simulink model "GridFormingConverter"  (R2023a)
settings: Solver=ode1be  StartTime=0.0  StopTime=simulationTime  FixedStep=gridInverter.vsm.samplingTime  MaxStep=gridInverter.vsm.samplingTime  RelTol=1e-3  AbsTol=1e-3
PreLoadFcn:
  | % Parameterize the model
  | GridFormingConverterInputParameters;
PostLoadFcn:
  | GridFormingConverterTestCondition;
undefined symbols (not defined in the file): base, DiscIntNeverNeededParam, grid, gridInverter, localSolverSampleTime, scrFactorRg, scrFactorXg, transformer, TransmissionLine
libraries: ee_lib x15, eeGeneralControl x15, nesl_utility x11, simulink x5, fl_lib x4, eeTransforms x4, eeSinGeneratorThreePhase x1, simulink_extras x1, eePowerMeasurement x1
(part 2 of 3)

== system GridFormingConverter/Grid-Forming Converter/Grid-Forming Converter Control/Current Limiting ==
  In Bus Element : Inport  PortName=measure  Element=Igd
  In Bus Element1 : Inport  PortName=measure  Element=Igq
  In Bus Element2 : Inport  Port=2  PortName=reactiveControl  Element=Vmd
  In Bus Element4 : Inport  Port=2  PortName=reactiveControl  Element=Vmq
  CurrentLimitingMethod : Subsystem  Variant=on  VariantControlMode=label  VariantControl=Choice  LabelModeActiveChoice=virimp
  Subtract : Sum  Inputs=+-
  Subtract1 : Sum  Inputs=-+
  Out Bus Element : Outport  PortName=currentLimiting  Element=Vmd
  Out Bus Element1 : Outport  PortName=currentLimiting  Element=Vmq
  Out Bus Element2 : Outport  PortName=currentLimiting  Element=Idmax
  Out Bus Element3 : Outport  PortName=currentLimiting  Element=Iqmax
  wires:
  In Bus Element2/1 -> Subtract/1
  In Bus Element1/1 -> CurrentLimitingMethod/2(Igq)
  In Bus Element4/1 -> Subtract1/2
  Subtract/1 -> Out Bus Element/1
  Subtract1/1 -> Out Bus Element1/1
  In Bus Element/1 -> CurrentLimitingMethod/1(Igd)  "Q"
  CurrentLimitingMethod/1(delVd) -> Subtract/2
  CurrentLimitingMethod/2(delVq) -> Subtract1/1
  CurrentLimitingMethod/3(Idmax) -> Out Bus Element2/1
  CurrentLimitingMethod/4(Iqmax) -> Out Bus Element3/1

== system GridFormingConverter/Grid-Forming Converter/Grid-Forming Converter Control/Grid Voltage Reactive Power Support ==
  In Bus Element1 : Inport  PortName=measure  Element=Vgd
  In Bus Element3 : Inport  PortName=measure  Element=Vgq
  In Bus Element2 : Inport  PortName=measure  Element=Igd
  In Bus Element4 : Inport  PortName=measure  Element=Igq
  PrefInput : Inport  Port=2
  QrefInput : Inport  Port=3
  Modifying Active Power Reference : Subsystem
  Modifying Reactive Power Reference : Subsystem
  Rate Transition{,1..5} (6 alike) : RateTransition
  Pref : Outport
  Qref : Outport  Port=2
  wires:
  PrefInput/1 -> Modifying Active Power Reference/1(PrefInput)
  In Bus Element2/1 -> Modifying Active Power Reference/3(Igd)
  In Bus Element4/1 -> Modifying Active Power Reference/4(Igq)
  In Bus Element3/1 -> Rate Transition2/1
  QrefInput/1 -> Rate Transition3/1
  Modifying Reactive Power Reference/1(PrefNew) -> Rate Transition4/1
  Modifying Reactive Power Reference/2(QrefNew) -> Rate Transition5/1
  In Bus Element1/1 -> Rate Transition/1
  Modifying Active Power Reference/1(Pref) -> Rate Transition1/1
  Rate Transition2/1 -> Modifying Reactive Power Reference/2(Vgq)
  Rate Transition3/1 -> Modifying Reactive Power Reference/3(Qref)
  Rate Transition1/1 -> Modifying Reactive Power Reference/4(Pref)
  Rate Transition4/1 -> Pref/1
  Rate Transition5/1 -> Qref/1
  Rate Transition/1 -> Modifying Reactive Power Reference/1(Vgd), Modifying Active Power Reference/2(Vd)

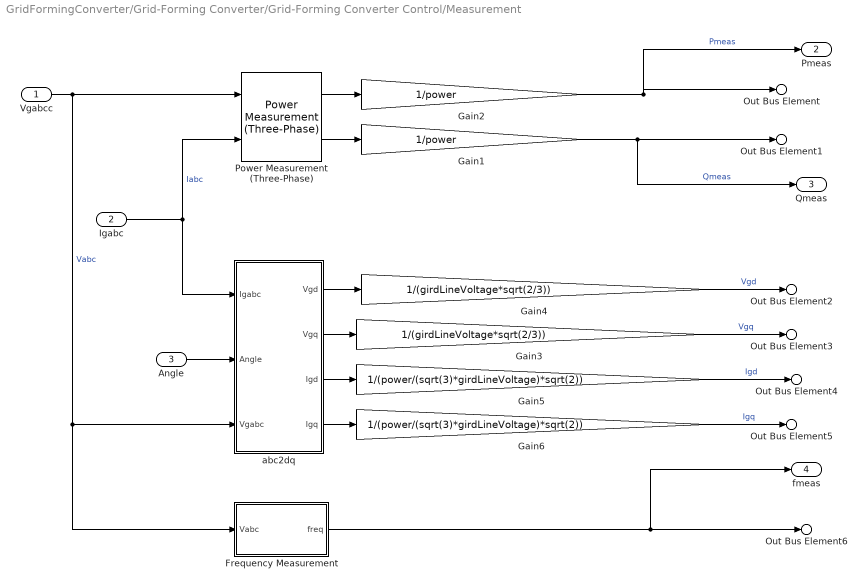
== system GridFormingConverter/Grid-Forming Converter/Grid-Forming Converter Control/Measurement ==
  Vgabcc : Inport
  Igabc : Inport  Port=2
  Angle : Inport  Port=3
  Frequency Measurement : Subsystem
  Gain1 : Gain  Gain=1/power
  Gain2 : Gain  Gain=1/power
  Gain3 : Gain  Gain=1/(girdLineVoltage*sqrt(2/3))
  Gain4 : Gain  Gain=1/(girdLineVoltage*sqrt(2/3))
  Gain5 : Gain  Gain=1/(power/(sqrt(3)*girdLineVoltage)*sqrt(2))
  Gain6 : Gain  Gain=1/(power/(sqrt(3)*girdLineVoltage)*sqrt(2))
  Power Measurement (Three-Phase) : eePowerMeasurement/Power Measurement (Three-Phase)  LabelModeActiveChoice=Continuous  F=powerFreq  K=[1]  Seq=Positive  Ts=measSampleTime
  abc2dq : Subsystem
  Out Bus Element : Outport  PortName=measure  Element=P
  Out Bus Element1 : Outport  PortName=measure  Element=Q
  Out Bus Element2 : Outport  PortName=measure  Element=Vgd
  Out Bus Element3 : Outport  PortName=measure  Element=Vgq
  Out Bus Element4 : Outport  PortName=measure  Element=Igd
  Out Bus Element5 : Outport  PortName=measure  Element=Igq
  Out Bus Element6 : Outport  PortName=measure  Element=fgrid
  Pmeas : Outport  Port=2
  Qmeas : Outport  Port=3
  fmeas : Outport  Port=4
  wires:
  Vgabcc/1 -> abc2dq/3(Vgabc), Frequency Measurement/1(Vabc), Power Measurement (Three-Phase)/1  "Vabc"
  Angle/1 -> abc2dq/2(Angle)
  Power Measurement (Three-Phase)/1 -> Gain2/1
  Igabc/1 -> abc2dq/1(Igabc), Power Measurement (Three-Phase)/2  "Iabc"
  Power Measurement (Three-Phase)/2 -> Gain1/1
  Gain2/1 -> Pmeas/1, Out Bus Element/1  "Pmeas"
  Gain1/1 -> Qmeas/1, Out Bus Element1/1  "Qmeas"
  abc2dq/1(Vgd) -> Gain4/1
  abc2dq/2(Vgq) -> Gain3/1
  abc2dq/3(Igd) -> Gain5/1
  abc2dq/4(Igq) -> Gain6/1
  Gain3/1 -> Out Bus Element3/1  "Vgq"
  Gain4/1 -> Out Bus Element2/1  "Vgd"
  Gain5/1 -> Out Bus Element4/1  "Igd"
  Gain6/1 -> Out Bus Element5/1  "Igq"
  Frequency Measurement/1(freq) -> Out Bus Element6/1, fmeas/1

== system GridFormingConverter/Grid-Forming Converter/Grid-Forming Converter Control/Power Control ==
  note: Reactive Power Control
  note: Active Power Control
  In Bus Element2 : Inport  PortName=measure  Element=P
  In Bus Element3 : Inport  PortName=measure  Element=Q
  In Bus Element1 : Inport  PortName=measure  Element=fgrid
  Pref : Inport  Port=2
  Qref : Inport  Port=3
  ActivePowerControl : Subsystem  Variant=on  VariantControlMode=label  VariantControl=Choice  LabelModeActiveChoice=vsm
  ReactiveControl : Subsystem
  Out Bus Element : Outport  PortName=reactiveControl  Element=Vmd
  Out Bus Element1 : Outport  PortName=reactiveControl  Element=Vmq
  Out Bus Element6 : Outport  Port=2  PortName=activeControl  Element=angle
  Out Bus Element4 : Outport  Port=2  PortName=activeControl  Element=w
  angle : Outport  Port=3
  wires:
  ActivePowerControl/2(w) -> Out Bus Element4/1
  In Bus Element3/1 -> ReactiveControl/2(Qmeas)
  ActivePowerControl/1(Theta) -> angle/1, Out Bus Element6/1
  ReactiveControl/1(Vmd) -> Out Bus Element/1
  ReactiveControl/2(Vmq) -> Out Bus Element1/1
  Pref/1 -> ActivePowerControl/1(Pref)  "Q"
  Qref/1 -> ReactiveControl/1(Qref)  "Q"
  In Bus Element2/1 -> ActivePowerControl/2(Pmeas)
  In Bus Element1/1 -> ActivePowerControl/3(fgrid)

== system GridFormingConverter/Grid-Forming Converter/Grid-Forming Converter Control/VoltageCurrentControl ==
  In Bus Element : Inport  PortName=currentLimiting  Element=Vmd
  In Bus Element1 : Inport  PortName=currentLimiting  Element=Vmq
  In Bus Element6 : Inport  PortName=currentLimiting  Element=Idmax
  In Bus Element7 : Inport  PortName=currentLimiting  Element=Iqmax
  Bus Element In6 : Inport  Port=2  PortName=activeControl  Element=w
  Bus Element In1 : Inport  Port=2  PortName=activeControl  Element=angle
  In Bus Element2 : Inport  Port=3  PortName=measure  Element=Vgd
  In Bus Element3 : Inport  Port=3  PortName=measure  Element=Vgq
  In Bus Element4 : Inport  Port=3  PortName=measure  Element=Igd
  In Bus Element5 : Inport  Port=3  PortName=measure  Element=Igq
  Controller : Subsystem
  Modulation Signal : Subsystem
  mabc : Outport
  wires:
  Controller/2(Vq) -> Modulation Signal/2(Vq)
  Modulation Signal/1(mabc) -> mabc/1
  Controller/1(Vd) -> Modulation Signal/1(Vd)
  In Bus Element4/1 -> Controller/6(Id)
  In Bus Element5/1 -> Controller/7(Iq)
  In Bus Element6/1 -> Controller/8(Idmax)
  In Bus Element7/1 -> Controller/9(Iqmax)
  In Bus Element2/1 -> Controller/4(Vsd)
  In Bus Element3/1 -> Controller/5(Vsq)
  Bus Element In6/1 -> Controller/1(Angfreq)
  In Bus Element/1 -> Controller/2(Vgdref)
  In Bus Element1/1 -> Controller/3(Vgqref)
  Bus Element In1/1 -> Modulation Signal/3(Angle)

== system GridFormingConverter/Grid-Forming Converter/Grid-Forming Converter Power Circuit/Filter & Sensor ==
  Current Sensor (Three-Phase) : ee_lib/Sensors & Transducers/Current Sensor (Three-Phase)
  Electrical Reference1 : fl_lib/Electrical/Electrical Elements/Electrical Reference
  Low-Pass Filter (Discrete or Continuous)1 : eeGeneralControl/Low-Pass Filter (Discrete or Continuous)  K=1  T=1/(200*gridInverter.frequency)  B=inf  A=-inf  init_option=Specify as parameter  x0=0  Ts=gridInverter.controller.VoltageControlSampleTime
  Low-Pass Filter (Discrete or Continuous)2 : eeGeneralControl/Low-Pass Filter (Discrete or Continuous)  K=1  T=1/(200*gridInverter.frequency)  B=inf  A=-inf  init_option=Specify as parameter  x0=0  Ts=gridInverter.controller.VoltageControlSampleTime
  Neutral Port (Three-Phase) : ee_lib/Connectors & References/Neutral Port (Three-Phase)  G_parasitic=1e-12 1/Ohm
      settings: InternalSimscapePortConfiguration="{\"Bottom\":[],\"Left\":[{\"id\":\"N\",\"label\":\"~\",\"type\":\"foundation.electrical.three_phase\"}],\"Right\":[{\"id\":\"n\",\"label\":\"n\",\"type\":\"foundation.electrical.electrical\"}],\"Top\":[]}"
  PS-Simulink Converter : nesl_utility/PS-Simulink Converter  PhysicalDomain=network_engine_domain  SubClassName=ps_output  LeftPortType=input  RightPortType=output  PseudoPeriodic=off  Frequencies=[]  VectorFormat=inherit  Unit=inherit  AffineConversion=off
  PS-Simulink Converter1 : nesl_utility/PS-Simulink Converter  PhysicalDomain=network_engine_domain  SubClassName=ps_output  LeftPortType=input  RightPortType=output  PseudoPeriodic=off  Frequencies=[]  VectorFormat=inherit  Unit=inherit  AffineConversion=off
  Phase Voltage Sensor (Three-Phase) : ee_lib/Sensors & Transducers/Phase Voltage Sensor (Three-Phase)
  RLC (Three-Phase) : ee_lib/Passive/RLC Assemblies/RLC (Three-Phase)  component_structure=ee.enum.rlc.structure.SeriesRL  R=gridInverter.lineResistance Ohm  L=gridInverter.L H  C=1e-6 F  R_parasitic=0 Ohm  G_parasitic=0 1/Ohm  IL_specify=off  IL_priority=High  IL=[0, 0, 0] A  IL_nominal_specify=off  IL_nominal_unit=A  IL_nominal_value=1  VC_specify=off  VC_priority=High  VC=[0, 0, 0] V  VC_nominal_specify=off  VC_nominal_unit=V  VC_nominal_value=1
      settings: InternalSimscapePortConfiguration="{\"Bottom\":[],\"Left\":[{\"id\":\"N1\",\"label\":\"~1\",\"type\":\"foundation.electrical.three_phase\"}],\"Right\":[{\"id\":\"N2\",\"label\":\"~2\",\"type\":\"foundation.electrical.three_phase\"}],\"Top\":[]}"
  Inabc : PMIOPort  Side=Left
  Opabc : PMIOPort  Port=2  Side=Right
  Iabc : Outport
  Vabc : Outport  Port=2
  wires:
  PS-Simulink Converter1/1 -> Low-Pass Filter (Discrete or Continuous)1/1
  Low-Pass Filter (Discrete or Continuous)2/1 -> Iabc/1
  PS-Simulink Converter/1 -> Low-Pass Filter (Discrete or Continuous)2/1
  Low-Pass Filter (Discrete or Continuous)1/1 -> Vabc/1
  connections:
  PS-Simulink Converter1/LConn1 -- Phase Voltage Sensor (Three-Phase)/RConn1
  Current Sensor (Three-Phase)/RConn2 -- RLC (Three-Phase)/LConn1
  Current Sensor (Three-Phase)/LConn1 -- Inabc/RConn1
  PS-Simulink Converter/LConn1 -- Current Sensor (Three-Phase)/RConn1
  Phase Voltage Sensor (Three-Phase)/LConn1 -- Opabc/RConn1 -- RLC (Three-Phase)/RConn1
  Phase Voltage Sensor (Three-Phase)/RConn2 -- Neutral Port (Three-Phase)/LConn1
  Electrical Reference1/LConn1 -- Neutral Port (Three-Phase)/RConn1

== system GridFormingConverter/Grid-Forming Converter/Grid-Forming Converter Control/Current Limiting/CurrentLimitingMethod ==
  Igd : Inport
  Igq : Inport  Port=2
  currentLimitAndVirtual : Subsystem  VariantControl=both
  currentSaturation : Subsystem  VariantControl=ctSat
  virtualImpedance : Subsystem  VariantControl=virimp
  delVd : Outport
  delVq : Outport  Port=2
  Idmax : Outport  Port=3
  Iqmax : Outport  Port=4

== system GridFormingConverter/Grid-Forming Converter/Grid-Forming Converter Control/Grid Voltage Reactive Power Support/Modifying Active Power Reference ==
  PrefInput : Inport
  Vd : Inport  Port=2
  Igd : Inport  Port=3
  Igq : Inport  Port=4
  AND : Logic  IconShape=distinctive  AllPortsSameDT=off  OutDataTypeStr=boolean
  Abs : Abs  SaturateOnIntegerOverflow=off
  Compare To Constant : simulink/Logic and Bit Operations/Compare To Constant  relop=<=  const=0.90  OutDataTypeStr=boolean
  Computing New Active Power Ref : Subsystem
  Math Function1 : Math  Operator=hypot
  Power Sign : Signum
  Product : Product
  Rate Transition1 : RateTransition
  Relay : Relay  OnSwitchValue=maxVICurrentLimit*0.96  OffSwitchValue=1
  Switch : Switch  Criteria=u2 > Threshold  SaturateOnIntegerOverflow=off  InputSameDT=off
  Pref : Outport
  wires:
  Computing New Active Power Ref/1(Pref) -> Switch/1
  Math Function1/1 -> Rate Transition1/1  "Is"
  Vd/1 -> Computing New Active Power Ref/2(Vd), Compare To Constant/1
  PrefInput/1 -> Power Sign/1, Switch/3
  Igd/1 -> Math Function1/2
  Switch/1 -> Abs/1
  Abs/1 -> Product/1
  Power Sign/1 -> Product/2
  Product/1 -> Pref/1
  Relay/1 -> AND/2
  AND/1 -> Switch/2
  Compare To Constant/1 -> AND/1
  Igq/1 -> Computing New Active Power Ref/1(Iq), Math Function1/1
  Rate Transition1/1 -> Relay/1

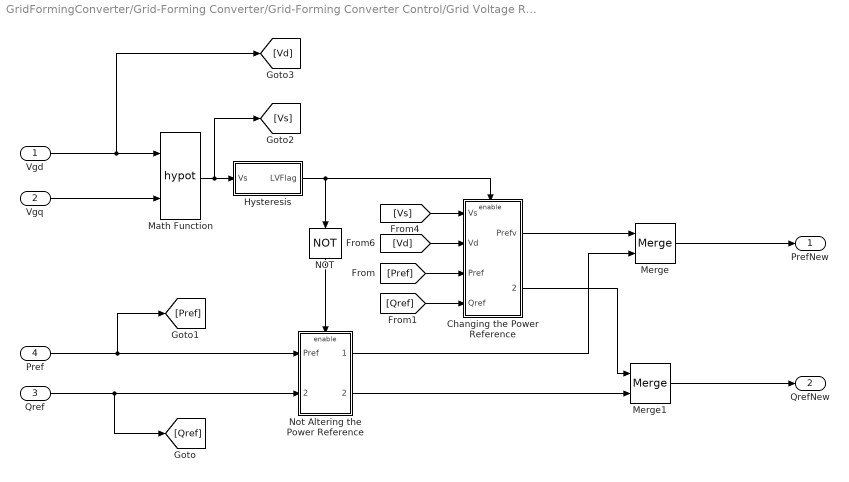
== system GridFormingConverter/Grid-Forming Converter/Grid-Forming Converter Control/Grid Voltage Reactive Power Support/Modifying Reactive Power Reference ==
  Vgd : Inport
  Vgq : Inport  Port=2
  Qref : Inport  Port=3
  Pref : Inport  Port=4
  Changing the Power Reference : Subsystem
  Hysteresis : Subsystem
  Math Function : Math  Operator=hypot
  Merge : Merge
  Merge1 : Merge
  NOT : Logic  Operator=NOT  IconShape=distinctive  AllPortsSameDT=off  OutDataTypeStr=boolean
  Not Altering the Power Reference : Subsystem
  PrefNew : Outport
  QrefNew : Outport  Port=2
  wires:
  Vgd/1 -> [Vd], Math Function/1
  Not Altering the Power Reference/2(Qrefv) -> Merge1/2
  Math Function/1 -> Hysteresis/1(Vs), [Vs]
  [Vs] -> Changing the Power Reference/1(Vs)
  Not Altering the Power Reference/1(Prefv) -> Merge/2
  Changing the Power Reference/1(Prefv) -> Merge/1
  NOT/1 -> Not Altering the Power Reference/Enable
  Qref/1 -> Not Altering the Power Reference/2(Qref), [Qref]
  Hysteresis/1(LVFlag) -> Changing the Power Reference/Enable, NOT/1
  [Vd] -> Changing the Power Reference/2(Vd)
  Changing the Power Reference/2(Qrefv) -> Merge1/1
  Vgq/1 -> Math Function/2
  Pref/1 -> Not Altering the Power Reference/1(Pref), [Pref]
  Merge1/1 -> QrefNew/1
  Merge/1 -> PrefNew/1
  [Pref] -> Changing the Power Reference/3(Pref)
  [Qref] -> Changing the Power Reference/4(Qref)

== system GridFormingConverter/Grid-Forming Converter/Grid-Forming Converter Control/Measurement/Frequency Measurement ==
  Vabc : Inport
  Convert To PU : Gain  Gain=1/powerFreq
  Frequency Measurement : Subsystem  TreatAsAtomicUnit=on  SystemSampleTime=sampleTime  mask{initialFrequency=powerFreq, sampleTime=activePowerSampleTime}
      mask prompts: initialFrequency "Initial frequency in Hz"; sampleTime "Sample time in sec"
      mask DialogControl Container7 Prompt: General
  Low-Pass Filter : eeGeneralControl/Low-Pass Filter (Discrete or Continuous)  K=1  T=freqMeasTimeConst  B=inf  A=-inf  init_option=Inherited from block input  x0=0  Ts=-1
  freq : Outport
  wires:
  Low-Pass Filter/1 -> Convert To PU/1  "Freq"
  Frequency Measurement/1(Freq) -> Low-Pass Filter/1
  Convert To PU/1 -> freq/1
  Vabc/1 -> Frequency Measurement/1(abc)

== system GridFormingConverter/Grid-Forming Converter/Grid-Forming Converter Control/Measurement/abc2dq ==
  Igabc : Inport
  Angle : Inport  Port=2
  Vgabc : Inport  Port=3
  Supply Current to dq : Subsystem
  Supply Voltage  to dq : Subsystem
  Vgd : Outport
  Vgq : Outport  Port=2
  Igd : Outport  Port=3
  Igq : Outport  Port=4
  wires:
  Angle/1 -> Supply Voltage  to dq/1(Angle), Supply Current to dq/2(Angle)
  Vgabc/1 -> Supply Voltage  to dq/2(abc)
  Igabc/1 -> Supply Current to dq/1(abc)
  Supply Current to dq/1(Igd) -> Igd/1  "Id"
  Supply Current to dq/2(Igq) -> Igq/1  "Iq"
  Supply Voltage  to dq/1(Vgd) -> Vgd/1  "Vgd"
  Supply Voltage  to dq/2(Vgq) -> Vgq/1  "Vgq"

== system GridFormingConverter/Grid-Forming Converter/Grid-Forming Converter Control/Power Control/ActivePowerControl ==
  Pref : Inport
  Pmeas : Inport  Port=2
  fgrid : Inport  Port=3
  droopControl : Subsystem  VariantControl=droop
  vsmControl : Subsystem  VariantControl=vsm
  Theta : Outport
  w : Outport  Port=2

== system GridFormingConverter/Grid-Forming Converter/Grid-Forming Converter Control/Power Control/ReactiveControl ==
  note: Vs-delV
  Qref : Inport
  Qmeas : Inport  Port=2
  Constant : Constant  Value=voltreference
  Constant2 : Constant  Value=0
  Gain : Gain  Gain=QVoltDroop
  Low-Pass Filter (Discrete or Continuous) : eeGeneralControl/Low-Pass Filter (Discrete or Continuous)  K=1  T=QVoltFilterTC  B=inf  A=-inf  init_option=Specify as parameter  x0=0  Ts=activePowerSampleTime
  Product1 : Product
  Saturation1 : Saturate  UpperLimit=(dcBusVoltage/2)/(sqrt(2/3)*girdLineVoltage)  LowerLimit=-(dcBusVoltage/2)/(sqrt(2/3)*girdLineVoltage)
  Sum : Sum  Inputs=|+-
  Sum1 : Sum  Inputs=|++
  Vmd : Outport
  Vmq : Outport  Port=2
  wires:
  Sum/1 -> Gain/1
  Qmeas/1 -> Low-Pass Filter (Discrete or Continuous)/1
  Low-Pass Filter (Discrete or Continuous)/1 -> Sum/2
  Gain/1 -> Sum1/1
  Product1/1 -> Saturation1/1  "Q"
  Constant/1 -> Product1/2, Sum1/2
  Constant2/1 -> Vmq/1
  Sum1/1 -> Product1/1
  Qref/1 -> Sum/1
  Saturation1/1 -> Vmd/1

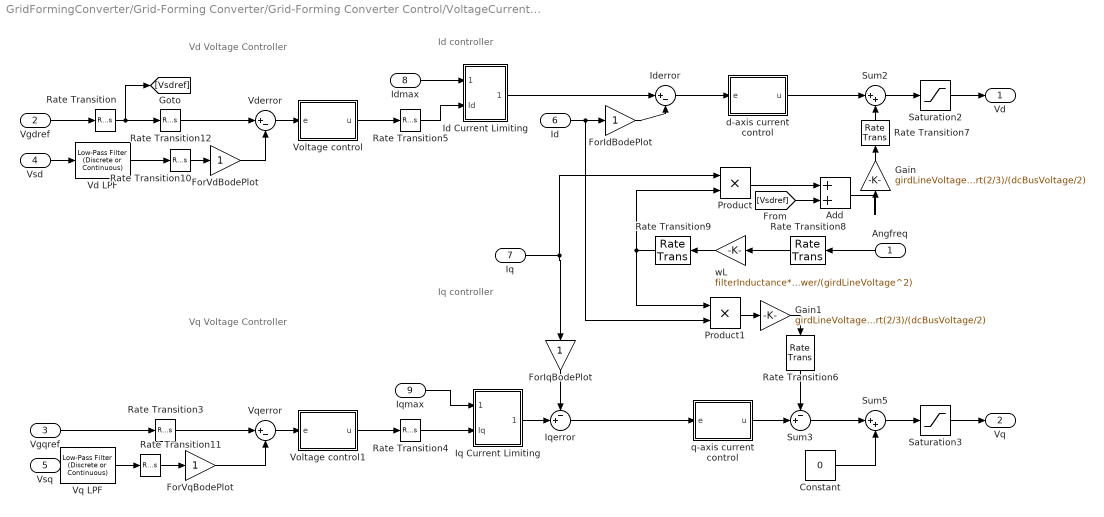
== system GridFormingConverter/Grid-Forming Converter/Grid-Forming Converter Control/VoltageCurrentControl/Controller ==
  note: Id controller
  note: Vd Voltage Controller
  note: Iq controller
  note: Vq Voltage Controller
  Angfreq : Inport
  Vgdref : Inport  Port=2
  Vgqref : Inport  Port=3
  Vsd : Inport  Port=4
  Vsq : Inport  Port=5
  Id : Inport  Port=6
  Iq : Inport  Port=7
  Idmax : Inport  Port=8
  Iqmax : Inport  Port=9
  Add : Sum
  Constant : Constant  Value=0  SampleTime=currentControlTs
  ForIdBodePlot : Gain
  ForIqBodePlot : Gain
  ForVdBodePlot : Gain
  ForVqBodePlot : Gain
  Gain : Gain  Gain=girdLineVoltage*sqrt(2/3)/(dcBusVoltage/2)
  Gain1 : Gain  Gain=girdLineVoltage*sqrt(2/3)/(dcBusVoltage/2)
  Id Current Limiting : Subsystem
  Iderror : Sum  Inputs=|+-
  Iq Current Limiting : Subsystem
  Iqerror : Sum  Inputs=-+|
  Product : Product
  Product1 : Product
  Rate Transition{,3..12} (11 alike) : RateTransition
  Saturation2 : Saturate  UpperLimit=4  LowerLimit=-3
  Saturation3 : Saturate  UpperLimit=3  LowerLimit=-3
  Sum2 : Sum  Inputs=|++
  Sum3 : Sum  Inputs=-+|
  Sum5 : Sum  Inputs=|++
  Vd LPF : eeGeneralControl/Low-Pass Filter (Discrete or Continuous)  K=1  T=vdvqLPFTimeConst  B=inf  A=-inf  init_option=Specify as parameter  x0=0  Ts=voltControlTs
  Vderror : Sum  Inputs=|+-
  Voltage control : Subsystem
  Voltage control1 : Subsystem
  Vq LPF : eeGeneralControl/Low-Pass Filter (Discrete or Continuous)  K=1  T=vdvqLPFTimeConst  B=inf  A=-inf  init_option=Inherited from block input  x0=0  Ts=voltControlTs
  Vqerror : Sum  Inputs=|+-
  d-axis current control : Subsystem
  q-axis current control : Subsystem
  wL : Gain  Gain=filterInductance*power/(girdLineVoltage^2)
  Vd : Outport  VectorParamsAs1DForOutWhenUnconnected=off
  Vq : Outport  Port=2  VectorParamsAs1DForOutWhenUnconnected=off
  wires:
  Iqerror/1 -> q-axis current control/1(e)
  wL/1 -> Rate Transition9/1
  Iq/1 -> ForIqBodePlot/1, Product/1
  Angfreq/1 -> Rate Transition8/1
  Constant/1 -> Sum5/2
  Iderror/1 -> d-axis current control/1(e)
  Saturation3/1 -> Vq/1
  Saturation2/1 -> Vd/1
  Product1/1 -> Gain1/1
  Product/1 -> Add/1
  d-axis current control/1(u) -> Sum2/1
  Sum2/1 -> Saturation2/1
  q-axis current control/1(u) -> Sum3/2
  Sum3/1 -> Sum5/1
  Sum5/1 -> Saturation3/1
  Vsq/1 -> Vq LPF/1
  Id/1 -> Product1/2, ForIdBodePlot/1
  Vderror/1 -> Voltage control/1(e)
  Iqmax/1 -> Iq Current Limiting/1(Imax)
  Vgqref/1 -> Rate Transition3/1
  Vqerror/1 -> Voltage control1/1(e)
  Gain1/1 -> Rate Transition6/1
  [Vsdref] -> Add/2
  Add/1 -> Gain/1
  Gain/1 -> Rate Transition7/1
  Voltage control/1(u) -> Rate Transition5/1
  Idmax/1 -> Id Current Limiting/1(Imax)
  Iq Current Limiting/1(Iqref) -> Iqerror/2
  Voltage control1/1(u) -> Rate Transition4/1
  Vsd/1 -> Vd LPF/1
  ForIdBodePlot/1 -> Iderror/2
  ForIqBodePlot/1 -> Iqerror/1
  Id Current Limiting/1(Idref) -> Iderror/1
  Vgdref/1 -> Rate Transition/1
  Rate Transition/1 -> [Vsdref], Rate Transition12/1
  Rate Transition3/1 -> Vqerror/1
  Rate Transition4/1 -> Iq Current Limiting/2(Iq)
  Rate Transition5/1 -> Id Current Limiting/2(Id)
  Rate Transition6/1 -> Sum3/1
  Rate Transition7/1 -> Sum2/2
  Rate Transition8/1 -> wL/1
  Vq LPF/1 -> Rate Transition11/1
  Rate Transition9/1 -> Product/2, Product1/1
  ForVdBodePlot/1 -> Vderror/2
  ForVqBodePlot/1 -> Vqerror/2
  Vd LPF/1 -> Rate Transition10/1
  Rate Transition10/1 -> ForVdBodePlot/1
  Rate Transition11/1 -> ForVqBodePlot/1
  Rate Transition12/1 -> Vderror/1

== system GridFormingConverter/Grid-Forming Converter/Grid-Forming Converter Control/VoltageCurrentControl/Modulation Signal ==
  Vd : Inport
  Vq : Inport  Port=2
  Angle : Inport  Port=3
  Constant : Constant  Value=0
  Inverse Park Transform : eeTransforms/Inverse Park Transform  AxisAlignment=D-axis  PowerInvariant=off
  Mux1 : Mux  Inputs=3
  Saturation2 : Saturate  UpperLimit=1  LowerLimit=-1
  mabc : Outport  VectorParamsAs1DForOutWhenUnconnected=off
  wires:
  Inverse Park Transform/1 -> Saturation2/1
  Mux1/1 -> Inverse Park Transform/1
  Saturation2/1 -> mabc/1
  Constant/1 -> Mux1/3
  Vd/1 -> Mux1/1
  Angle/1 -> Inverse Park Transform/2
  Vq/1 -> Mux1/2

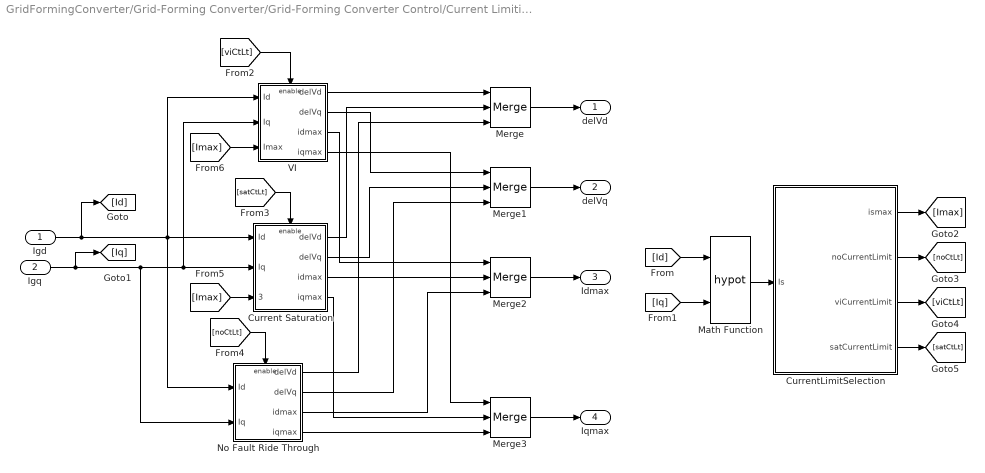
== system GridFormingConverter/Grid-Forming Converter/Grid-Forming Converter Control/Current Limiting/CurrentLimitingMethod/currentLimitAndVirtual ==
  Igd : Inport
  Igq : Inport  Port=2
  Current Saturation : Subsystem
  CurrentLimitSelection : Stateflow chart  TreatAsAtomicUnit=on
  Math Function : Math  Operator=hypot
  Merge{,1..3} (4 alike) : Merge  Inputs=3
  No Fault Ride Through : Subsystem
  VI : Subsystem
  delVd : Outport
  delVq : Outport  Port=2
  Idmax : Outport  Port=3
  Iqmax : Outport  Port=4
  wires:
  Merge2/1 -> Idmax/1
  Igq/1 -> Current Saturation/2(Iq), VI/2(Iq), No Fault Ride Through/2(Iq), [Iq]
  Merge1/1 -> delVq/1
  Igd/1 -> VI/1(Id), Current Saturation/1(Id), No Fault Ride Through/1(Id), [Id]
  No Fault Ride Through/1(delVd) -> Merge/3
  No Fault Ride Through/3(idmax) -> Merge2/3
  VI/1(delVd) -> Merge/1
  [Iq] -> Math Function/2
  [Id] -> Math Function/1
  Current Saturation/1(delVd) -> Merge/2
  Current Saturation/4(iqmax) -> Merge3/2
  Merge/1 -> delVd/1
  VI/2(delVq) -> Merge1/1
  Current Saturation/3(idmax) -> Merge2/2
  VI/4(iqmax) -> Merge3/1
  VI/3(idmax) -> Merge2/1
  No Fault Ride Through/4(iqmax) -> Merge3/3
  Current Saturation/2(delVq) -> Merge1/2
  Merge3/1 -> Iqmax/1
  No Fault Ride Through/2(delVq) -> Merge1/3
  Math Function/1 -> CurrentLimitSelection/1(Is)
  CurrentLimitSelection/1(ismax) -> [Imax]
  CurrentLimitSelection/2(noCurrentLimit) -> [noCtLt]
  CurrentLimitSelection/3(viCurrentLimit) -> [viCtLt]
  CurrentLimitSelection/4(satCurrentLimit) -> [satCtLt]
  [viCtLt] -> VI/Enable
  [satCtLt] -> Current Saturation/Enable
  [noCtLt] -> No Fault Ride Through/Enable
  [Imax] -> Current Saturation/3(Imaxsat)
  [Imax] -> VI/3(Imax)

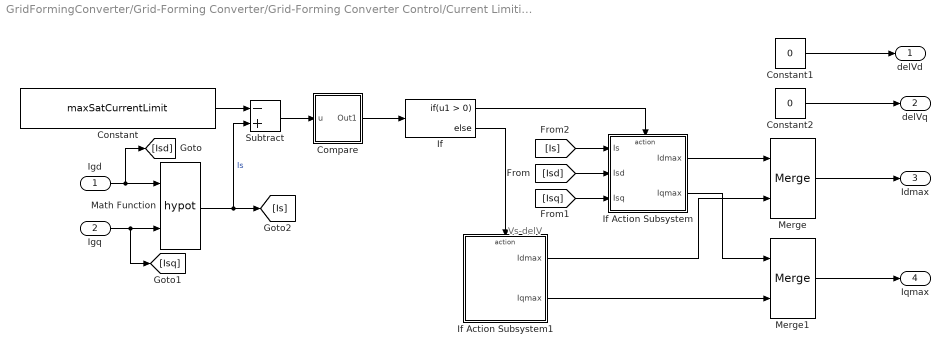
== system GridFormingConverter/Grid-Forming Converter/Grid-Forming Converter Control/Current Limiting/CurrentLimitingMethod/currentSaturation ==
  note: Vs-delV
  Igd : Inport
  Igq : Inport  Port=2
  Compare : Subsystem
  Constant : Constant  Value=maxSatCurrentLimit
  Constant1 : Constant  Value=0
  Constant2 : Constant  Value=0
  If : If
  If Action Subsystem : Subsystem  TreatAsAtomicUnit=on
  If Action Subsystem1 : Subsystem  TreatAsAtomicUnit=on
  Math Function : Math  Operator=hypot
  Merge : Merge
  Merge1 : Merge
  Subtract : Sum  Inputs=-+
  delVd : Outport
  delVq : Outport  Port=2
  Idmax : Outport  Port=3
  Iqmax : Outport  Port=4
  wires:
  Igd/1 -> [Isd], Math Function/1
  Igq/1 -> [Isq], Math Function/2
  Constant/1 -> Subtract/1
  Math Function/1 -> [Is], Subtract/2  "Is"
  If/1 -> If Action Subsystem/Action
  [Isd] -> If Action Subsystem/2(Isd)
  [Isq] -> If Action Subsystem/3(Isq)
  Subtract/1 -> Compare/1(u)
  Compare/1(Out1) -> If/1
  If/2 -> If Action Subsystem1/Action
  [Is] -> If Action Subsystem/1(Is)
  If Action Subsystem/1(Idmax) -> Merge/1
  If Action Subsystem1/1(Idmax) -> Merge/2
  If Action Subsystem/2(Iqmax) -> Merge1/1
  If Action Subsystem1/2(Iqmax) -> Merge1/2
  Constant2/1 -> delVq/1
  Constant1/1 -> delVd/1
  Merge/1 -> Idmax/1
  Merge1/1 -> Iqmax/1

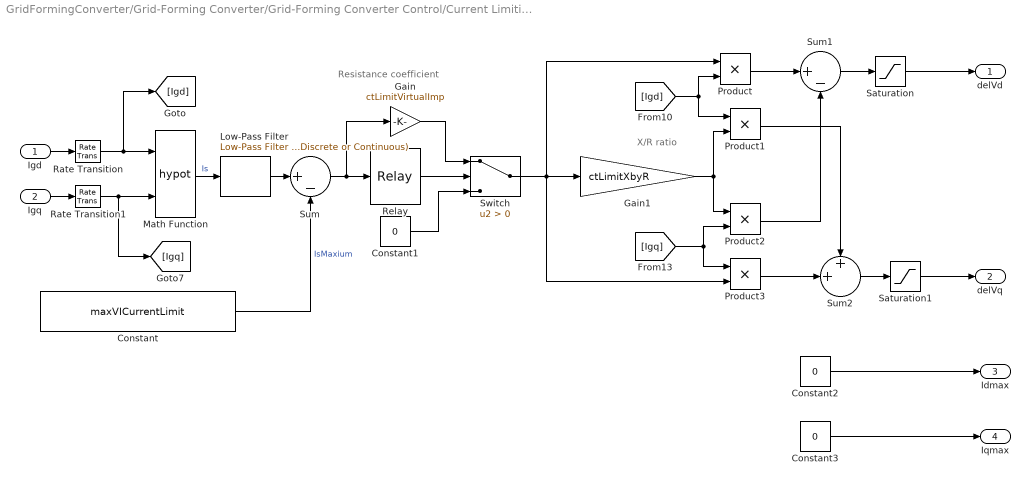
== system GridFormingConverter/Grid-Forming Converter/Grid-Forming Converter Control/Current Limiting/CurrentLimitingMethod/virtualImpedance ==
  note: X/R ratio
  note: Resistance coefficient
  Igd : Inport
  Igq : Inport  Port=2
  Constant : Constant  Value=maxVICurrentLimit
  Constant1 : Constant  Value=0
  Constant2 : Constant  Value=0
  Constant3 : Constant  Value=0
  Gain : Gain  Gain=ctLimitVirtualImp
  Gain1 : Gain  Gain=ctLimitXbyR
  Low-Pass Filter : eeGeneralControl/Low-Pass Filter (Discrete or Continuous)  K=1  T=currentVITimeConst  B=inf  A=-inf  init_option=Inherited from block input  x0=0  Ts=-1
  Math Function : Math  Operator=hypot
  Product{,1..3} (4 alike) : Product
  Rate Transition : RateTransition
  Rate Transition1 : RateTransition
  Relay : Relay  OnSwitchValue=0.01  OffSwitchValue=-0.05
  Saturation : Saturate  UpperLimit=1  LowerLimit=-1
  Saturation1 : Saturate  UpperLimit=1  LowerLimit=-1
  Sum : Sum  Inputs=|+-
  Sum1 : Sum  Inputs=|+-
  Sum2 : Sum  Inputs=++|
  Switch : Switch  Criteria=u2 > Threshold  SaturateOnIntegerOverflow=off  InputSameDT=off
  delVd : Outport
  delVq : Outport  Port=2
  Idmax : Outport  Port=3
  Iqmax : Outport  Port=4
  wires:
  Sum/1 -> Gain/1, Relay/1
  Igq/1 -> Rate Transition1/1
  Product1/1 -> Sum2/1
  Gain1/1 -> Product1/2, Product2/1
  Sum1/1 -> Saturation/1
  Product/1 -> Sum1/1
  Product2/1 -> Sum1/2
  Constant/1 -> Sum/2  "IsMaxium"
  Math Function/1 -> Low-Pass Filter/1  "Is"
  [Igq] -> Product3/1, Product2/2
  Switch/1 -> Gain1/1, Product3/2, Product/1
  [Igd] -> Product1/1, Product/2
  Constant2/1 -> Idmax/1
  Constant3/1 -> Iqmax/1
  Gain/1 -> Switch/1
  Constant1/1 -> Switch/3
  Igd/1 -> Rate Transition/1
  Saturation1/1 -> delVq/1
  Relay/1 -> Switch/2
  Saturation/1 -> delVd/1
  Low-Pass Filter/1 -> Sum/1
  Product3/1 -> Sum2/2
  Sum2/1 -> Saturation1/1
  Rate Transition/1 -> Math Function/1, [Igd]
  Rate Transition1/1 -> [Igq], Math Function/2

== system GridFormingConverter/Grid-Forming Converter/Grid-Forming Converter Control/Grid Voltage Reactive Power Support/Modifying Active Power Reference/Computing New Active Power Ref ==
  Iq : Inport
  Vd : Inport  Port=2
  Abs : Abs  SaturateOnIntegerOverflow=off
  Constant : Constant  Value=maxVICurrentLimit*0.96
  Constant1 : Constant  Value=0
  Product : Product
  Sqrt : Sqrt
  Square : Math  Operator=square
  Square1 : Math  Operator=square
  Subtract : Sum  Inputs=-+
  Switch : Switch  Criteria=u2 > Threshold  Threshold=1.15  SaturateOnIntegerOverflow=off  InputSameDT=off
  Pref : Outport
  wires:
  Constant/1 -> Square1/1
  Switch/1 -> Product/2
  Square/1 -> Subtract/1
  Square1/1 -> Subtract/2
  Vd/1 -> Product/1
  Sqrt/1 -> Abs/1
  Iq/1 -> Square/1
  Product/1 -> Pref/1
  Subtract/1 -> Switch/2, Sqrt/1
  Constant1/1 -> Switch/3
  Abs/1 -> Switch/1

== system GridFormingConverter/Grid-Forming Converter/Grid-Forming Converter Control/Grid Voltage Reactive Power Support/Modifying Reactive Power Reference/Changing the Power Reference ==
  Vs : Inport
  Vd : Inport  Port=2
  Pref : Inport  Port=3
  Qref : Inport  Port=4
  Enable : EnablePort
  ActivePowerReference : Subsystem
  Constant1 : Constant  Value=voltreference*0.96
  Estimate Id for Given Iq : Subsystem
  EstimateIqForReactivePower : Subsystem
  Max : MinMax  Function=max  Inputs=2
  ReactivePowerReference : Subsystem
  Prefv : Outport
  Qrefv : Outport  Port=2
  wires:
  EstimateIqForReactivePower/1(Iq) -> Estimate Id for Given Iq/1(Iq), ReactivePowerReference/2(Iq)
  Constant1/1 -> EstimateIqForReactivePower/1(Vmin)
  Vs/1 -> ActivePowerReference/2(Vd), EstimateIqForReactivePower/3(Vs), ReactivePowerReference/1(Vd)
  Estimate Id for Given Iq/1(Id) -> ActivePowerReference/1(Id)
  Pref/1 -> ActivePowerReference/3(Pref)
  ActivePowerReference/1(PrefNew) -> Prefv/1
  ReactivePowerReference/1(QrefNew) -> Max/1
  Max/1 -> Qrefv/1
  Qref/1 -> Max/2
  Vd/1 -> EstimateIqForReactivePower/2(Vd)

== system GridFormingConverter/Grid-Forming Converter/Grid-Forming Converter Control/Grid Voltage Reactive Power Support/Modifying Reactive Power Reference/Hysteresis ==
  Vs : Inport
  AND : Logic  IconShape=distinctive  AllPortsSameDT=off  OutDataTypeStr=boolean
  Compare To Constant : simulink/Logic and Bit Operations/Compare To Constant  relop=<  const=0.9  OutDataTypeStr=boolean
  Compare To Constant1 : simulink/Logic and Bit Operations/Compare To Constant  relop=<  const=0.95  OutDataTypeStr=boolean
  D Latch : simulink_extras/Flip Flops/D Latch
  OR : Logic  Operator=OR  IconShape=distinctive  AllPortsSameDT=off  OutDataTypeStr=boolean
  Terminator : Terminator
  LVFlag : Outport
  wires:
  Compare To Constant1/1 -> AND/1
  D Latch/1 -> AND/2
  AND/1 -> OR/1
  OR/1 -> LVFlag/1
  D Latch/2 -> Terminator/1
  Compare To Constant/1 -> D Latch/1, D Latch/2, OR/2
  Vs/1 -> Compare To Constant1/1, Compare To Constant/1

== system GridFormingConverter/Grid-Forming Converter/Grid-Forming Converter Control/Grid Voltage Reactive Power Support/Modifying Reactive Power Reference/Not Altering the Power Reference ==
  Pref : Inport
  Qref : Inport  Port=2
  Enable : EnablePort
  Prefv : Outport
  Qrefv : Outport  Port=2
  wires:
  Pref/1 -> Prefv/1
  Qref/1 -> Qrefv/1

== system GridFormingConverter/Grid-Forming Converter/Grid-Forming Converter Control/Measurement/Frequency Measurement/Frequency Measurement ==
  abc : Inport
  Constant : Constant
  Discrete-Time Integrator : DiscreteIntegrator  SampleTime=sampleTime  LimitOutput=on  ICPrevOutput=DiscIntNeverNeededParam  ICPrevScaledInput=DiscIntNeverNeededParam
  If : If  IfExpression=u1 > 0.9
  If Action Subsystem : Subsystem  TreatAsAtomicUnit=on
  If Action Subsystem1 : Subsystem  TreatAsAtomicUnit=on
  Merge : Merge
  Postive Sequence : Subsystem
  Freq : Outport
  wires:
  If/1 -> If Action Subsystem/Action
  If/2 -> If Action Subsystem1/Action
  Discrete-Time Integrator/1 -> If Action Subsystem/2(Time), If/1
  abc/1 -> Postive Sequence/1(abc)
  Constant/1 -> Discrete-Time Integrator/1
  If Action Subsystem/1(Freq) -> Merge/1
  If Action Subsystem1/1(Out1) -> Merge/2
  Merge/1 -> Freq/1
  Postive Sequence/1(posSeq) -> If Action Subsystem/1(V)

== system GridFormingConverter/Grid-Forming Converter/Grid-Forming Converter Control/Measurement/abc2dq/Supply Current to dq ==
  abc : Inport
  Angle : Inport  Port=2
  Demux : Demux  Outputs=3
  Park Transform : eeTransforms/Park Transform  AxisAlignment=D-axis  PowerInvariant=off
  Terminator : Terminator
  Igd : Outport  VectorParamsAs1DForOutWhenUnconnected=off
  Igq : Outport  Port=2  VectorParamsAs1DForOutWhenUnconnected=off
  wires:
  Demux/3 -> Terminator/1
  Park Transform/1 -> Demux/1
  Demux/2 -> Igq/1
  Demux/1 -> Igd/1
  abc/1 -> Park Transform/1
  Angle/1 -> Park Transform/2

== system GridFormingConverter/Grid-Forming Converter/Grid-Forming Converter Control/Measurement/abc2dq/Supply Voltage  to dq ==
  Angle : Inport
  abc : Inport  Port=2
  Demux : Demux  Outputs=3
  Park Transform : eeTransforms/Park Transform  AxisAlignment=D-axis  PowerInvariant=off
  Terminator : Terminator
  Vgd : Outport  VectorParamsAs1DForOutWhenUnconnected=off
  Vgq : Outport  Port=2  VectorParamsAs1DForOutWhenUnconnected=off
  wires:
  Demux/3 -> Terminator/1
  Park Transform/1 -> Demux/1
  Demux/2 -> Vgq/1
  Demux/1 -> Vgd/1
  abc/1 -> Park Transform/1
  Angle/1 -> Park Transform/2

== system GridFormingConverter/Grid-Forming Converter/Grid-Forming Converter Control/Power Control/ActivePowerControl/droopControl ==
  Pref : Inport
  Pmeas : Inport  Port=2
  fgrid : Inport  Port=3
  Add : Sum  Inputs=+-
  Constant : Constant
  Constant5 : Constant  Value=pi/2
  Gain : Gain  Gain=powerFreq*2*pi
  Integrator with Wrapped State (Discrete or Continuous) : eeGeneralControl/Integrator with Wrapped State (Discrete or Continuous)  LabelModeActiveChoice=Discrete  WrappedStateUpperValue=2*pi  WrappedStateLowerValue=0  x0=0  Ts=activePowerSampleTime
      settings: LibrarySourceBlock=|
      | ee_sl_lib/General Control/Integrator with
      | Wrapped State
      | (Discrete or Continuous)
  Lead-Lag (Discrete or Continuous) : eeGeneralControl/Lead-Lag (Discrete or Continuous)  T1=droopT1  T2=droopT2  B=inf  A=-inf  init_option=Inherited from block input  x0=0  Ts=activePowerSampleTime
      settings: LibrarySourceBlock=|
      | ee_sl_lib/General Control/Lead-Lag
      | (Discrete or Continuous)
  Low-Pass Filter (Discrete or Continuous) : eeGeneralControl/Low-Pass Filter (Discrete or Continuous)  K=1  T=droopTC  B=inf  A=-inf  init_option=Specify as parameter  x0=0  Ts=activePowerSampleTime
  Sum : Sum  Inputs=|-+
  Sum1 : Sum  Inputs=|-+
  Terminator : Terminator
  mp : Gain  Gain=droopSlope
  Theta : Outport
  w : Outport  Port=2
  wires:
  Low-Pass Filter (Discrete or Continuous)/1 -> Sum1/1
  mp/1 -> Low-Pass Filter (Discrete or Continuous)/1
  Sum/1 -> mp/1
  Pmeas/1 -> Lead-Lag (Discrete or Continuous)/1
  Add/1 -> Theta/1
  Constant5/1 -> Add/2
  Pref/1 -> Sum/1
  Gain/1 -> Integrator with Wrapped State (Discrete or Continuous)/1, w/1
  Lead-Lag (Discrete or Continuous)/1 -> Sum/2
  Integrator with Wrapped State (Discrete or Continuous)/1 -> Add/1
  Constant/1 -> Sum1/2
  Sum1/1 -> Gain/1
  fgrid/1 -> Terminator/1

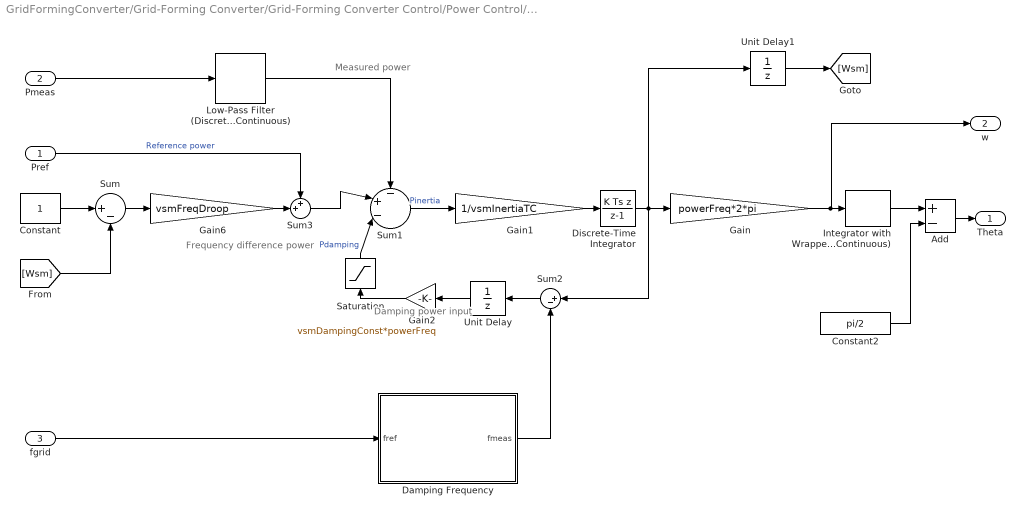
== system GridFormingConverter/Grid-Forming Converter/Grid-Forming Converter Control/Power Control/ActivePowerControl/vsmControl ==
  note: Measured power
  note: Frequency difference power
  note: Damping power input
  Pref : Inport
  Pmeas : Inport  Port=2
  fgrid : Inport  Port=3
  Add : Sum  Inputs=+-
  Constant : Constant
  Constant2 : Constant  Value=pi/2
  Damping Frequency : Subsystem  Variant=on  VariantControlMode=label  VariantControl=Choice  LabelModeActiveChoice=freqMeas
  Discrete-Time Integrator : DiscreteIntegrator  IntegratorMethod=Integration: Backward Euler  InitialCondition=1  SampleTime=activePowerSampleTime  LimitOutput=on  UpperSaturationLimit=1.1  LowerSaturationLimit=0.9  ICPrevOutput=DiscIntNeverNeededParam  ICPrevScaledInput=DiscIntNeverNeededParam
  Gain : Gain  Gain=powerFreq*2*pi
  Gain1 : Gain  Gain=1/vsmInertiaTC
  Gain2 : Gain  Gain=vsmDampingConst*powerFreq
  Gain6 : Gain  Gain=vsmFreqDroop
  Integrator with Wrapped State (Discrete or Continuous) : eeGeneralControl/Integrator with Wrapped State (Discrete or Continuous)  LabelModeActiveChoice=Discrete  WrappedStateUpperValue=2*pi  WrappedStateLowerValue=0  x0=0  Ts=activePowerSampleTime
      settings: LibrarySourceBlock=|
      | ee_sl_lib/General Control/Integrator with
      | Wrapped State
      | (Discrete or Continuous)
  Low-Pass Filter (Discrete or Continuous) : eeGeneralControl/Low-Pass Filter (Discrete or Continuous)  K=1  T=vsmPmeasFilterTC  B=inf  A=-inf  init_option=Specify as parameter  x0=0  Ts=activePowerSampleTime
  Saturation : Saturate  UpperLimit=dampingPowerMaxLimit  LowerLimit=dampingPowerMinLimit
  Sum : Sum  Inputs=|+-
  Sum1 : Sum  Inputs=-+-|
  Sum2 : Sum  Inputs=|+-
  Sum3 : Sum  Inputs=++|
  Unit Delay : UnitDelay  SampleTime=-1  HasFrameUpgradeWarning=on
  Unit Delay1 : UnitDelay  SampleTime=-1  HasFrameUpgradeWarning=on
  Theta : Outport
  w : Outport  Port=2
  wires:
  Integrator with Wrapped State (Discrete or Continuous)/1 -> Add/1
  Sum1/1 -> Gain1/1  "Pinertia"
  Sum/1 -> Gain6/1
  Constant2/1 -> Add/2
  Add/1 -> Theta/1
  Pmeas/1 -> Low-Pass Filter (Discrete or Continuous)/1
  Discrete-Time Integrator/1 -> Gain/1, Unit Delay1/1, Sum2/1
  [Wsm] -> Sum/2
  Low-Pass Filter (Discrete or Continuous)/1 -> Sum1/1
  Pref/1 -> Sum3/1  "Reference power"
  Gain2/1 -> Saturation/1
  Sum3/1 -> Sum1/2
  Sum2/1 -> Unit Delay/1
  Gain1/1 -> Discrete-Time Integrator/1
  Gain/1 -> Integrator with Wrapped State (Discrete or Continuous)/1, w/1
  Unit Delay/1 -> Gain2/1
  Constant/1 -> Sum/1
  Unit Delay1/1 -> [Wsm]
  Saturation/1 -> Sum1/3  "Pdamping"
  Gain6/1 -> Sum3/2
  fgrid/1 -> Damping Frequency/1(fref)
  Damping Frequency/1(fmeas) -> Sum2/2

== system GridFormingConverter/Grid-Forming Converter/Grid-Forming Converter Control/VoltageCurrentControl/Controller/Id Current Limiting ==
  Imax : Inport
  Id : Inport  Port=2
  Abs : Abs  SaturateOnIntegerOverflow=off
  Rate Transition : RateTransition
  Switch : Switch  Criteria=u2 > Threshold  SaturateOnIntegerOverflow=off  InputSameDT=off
  Idref : Outport
  wires:
  Id/1 -> Rate Transition/1
  Abs/1 -> Switch/2
  Imax/1 -> Abs/1, Switch/1
  Switch/1 -> Idref/1
  Rate Transition/1 -> Switch/3

== system GridFormingConverter/Grid-Forming Converter/Grid-Forming Converter Control/VoltageCurrentControl/Controller/Iq Current Limiting ==
  Imax : Inport
  Iq : Inport  Port=2
  Abs : Abs  SaturateOnIntegerOverflow=off
  Switch : Switch  Criteria=u2 > Threshold  SaturateOnIntegerOverflow=off  InputSameDT=off
  Iqref : Outport
  wires:
  Iq/1 -> Switch/3
  Abs/1 -> Switch/2
  Imax/1 -> Abs/1, Switch/1
  Switch/1 -> Iqref/1

== system GridFormingConverter/Grid-Forming Converter/Grid-Forming Converter Control/VoltageCurrentControl/Controller/Voltage control ==
  e : Inport
  Discrete-Time Integrator : DiscreteIntegrator  IntegratorMethod=Integration: Backward Euler  SampleTime=voltControlTs  LimitOutput=on  UpperSaturationLimit=VdMaxCt  LowerSaturationLimit=VdMinCt  ICPrevOutput=DiscIntNeverNeededParam  ICPrevScaledInput=DiscIntNeverNeededParam
  Ki : Gain  Gain=VdIGain
  Kp : Gain  Gain=vdPGain
  Limit : Saturate  UpperLimit=VdMaxCt  LowerLimit=VdMinCt
  Sum7 : Sum  Inputs=|++
  u : Outport  VectorParamsAs1DForOutWhenUnconnected=off
  wires:
  Discrete-Time Integrator/1 -> Sum7/2
  Kp/1 -> Sum7/1
  Limit/1 -> u/1
  Ki/1 -> Discrete-Time Integrator/1
  Sum7/1 -> Limit/1
  e/1 -> Kp/1, Ki/1

== system GridFormingConverter/Grid-Forming Converter/Grid-Forming Converter Control/VoltageCurrentControl/Controller/Voltage control1 ==
  e : Inport
  Discrete-Time Integrator : DiscreteIntegrator  IntegratorMethod=Integration: Backward Euler  SampleTime=voltControlTs  LimitOutput=on  UpperSaturationLimit=VqMaxCt  LowerSaturationLimit=VqMinCt  ICPrevOutput=DiscIntNeverNeededParam  ICPrevScaledInput=DiscIntNeverNeededParam
  Ki : Gain  Gain=VqIGain
  Kp : Gain  Gain=VqPGain
  Limit : Saturate  UpperLimit=VqMaxCt  LowerLimit=VqMinCt
  Sum7 : Sum  Inputs=|++
  u : Outport  VectorParamsAs1DForOutWhenUnconnected=off
  wires:
  Discrete-Time Integrator/1 -> Sum7/2
  Sum7/1 -> Limit/1
  e/1 -> Ki/1, Kp/1
  Kp/1 -> Sum7/1
  Ki/1 -> Discrete-Time Integrator/1
  Limit/1 -> u/1

== system GridFormingConverter/Grid-Forming Converter/Grid-Forming Converter Control/VoltageCurrentControl/Controller/d-axis current control ==
  e : Inport
  Discrete-Time Integrator : DiscreteIntegrator  IntegratorMethod=Integration: Backward Euler  SampleTime=currentControlTs  LimitOutput=on  UpperSaturationLimit=4  LowerSaturationLimit=-4  ICPrevOutput=DiscIntNeverNeededParam  ICPrevScaledInput=DiscIntNeverNeededParam
  Ki : Gain  Gain=IdIGain
  Kp : Gain  Gain=IdPGain
  Limit : Saturate  UpperLimit=4  LowerLimit=-4
  Sum7 : Sum  Inputs=|++
  u : Outport  VectorParamsAs1DForOutWhenUnconnected=off
  wires:
  Discrete-Time Integrator/1 -> Sum7/2
  Sum7/1 -> Limit/1
  e/1 -> Ki/1, Kp/1
  Kp/1 -> Sum7/1
  Limit/1 -> u/1
  Ki/1 -> Discrete-Time Integrator/1

== system GridFormingConverter/Grid-Forming Converter/Grid-Forming Converter Control/VoltageCurrentControl/Controller/q-axis current control ==
  e : Inport
  Discrete-Time Integrator : DiscreteIntegrator  IntegratorMethod=Integration: Backward Euler  SampleTime=currentControlTs  LimitOutput=on  UpperSaturationLimit=3  LowerSaturationLimit=-3  ICPrevOutput=DiscIntNeverNeededParam  ICPrevScaledInput=DiscIntNeverNeededParam
  Ki : Gain  Gain=IqIGain
  Kp : Gain  Gain=IqPGain
  Limit : Saturate  UpperLimit=3  LowerLimit=-3
  Sum7 : Sum  Inputs=|++
  u : Outport  VectorParamsAs1DForOutWhenUnconnected=off
  wires:
  Ki/1 -> Discrete-Time Integrator/1
  Kp/1 -> Sum7/1
  e/1 -> Kp/1, Ki/1
  Sum7/1 -> Limit/1
  Limit/1 -> u/1
  Discrete-Time Integrator/1 -> Sum7/2

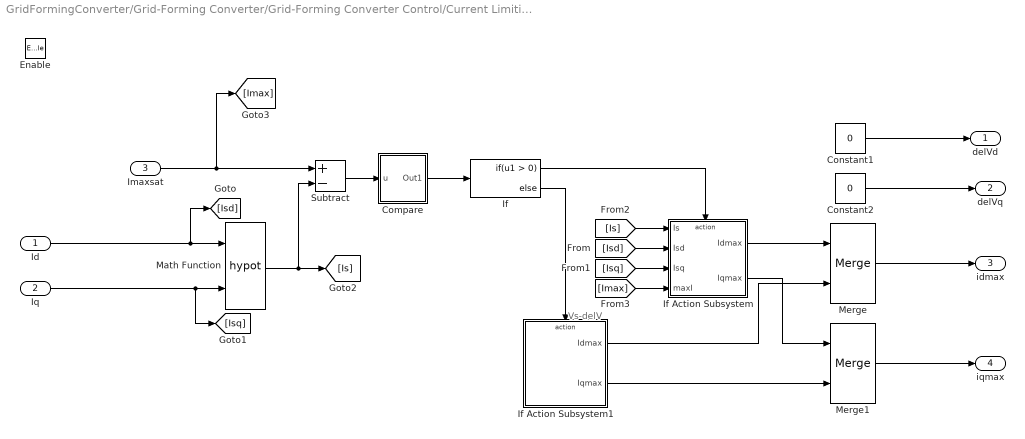
== system GridFormingConverter/Grid-Forming Converter/Grid-Forming Converter Control/Current Limiting/CurrentLimitingMethod/currentLimitAndVirtual/Current Saturation ==
  note: Vs-delV
  Id : Inport
  Iq : Inport  Port=2
  Imaxsat : Inport  Port=3
  Enable : EnablePort
  Compare : Subsystem
  Constant1 : Constant  Value=0
  Constant2 : Constant  Value=0
  If : If
  If Action Subsystem : Subsystem  TreatAsAtomicUnit=on
  If Action Subsystem1 : Subsystem  TreatAsAtomicUnit=on
  Math Function : Math  Operator=hypot
  Merge : Merge
  Merge1 : Merge
  Subtract : Sum  Inputs=+-
  delVd : Outport
  delVq : Outport  Port=2
  idmax : Outport  Port=3
  iqmax : Outport  Port=4
  wires:
  Iq/1 -> [Isq], Math Function/2
  If/1 -> If Action Subsystem/Action
  If Action Subsystem1/1(Idmax) -> Merge/2
  Constant2/1 -> delVq/1
  Math Function/1 -> [Is], Subtract/2
  If/2 -> If Action Subsystem1/Action
  If Action Subsystem/2(Iqmax) -> Merge1/1
  Subtract/1 -> Compare/1(u)
  Compare/1(Out1) -> If/1
  If Action Subsystem/1(Idmax) -> Merge/1
  [Is] -> If Action Subsystem/1(Is)
  Id/1 -> [Isd], Math Function/1
  If Action Subsystem1/2(Iqmax) -> Merge1/2
  Merge/1 -> idmax/1
  [Isd] -> If Action Subsystem/2(Isd)
  Constant1/1 -> delVd/1
  [Isq] -> If Action Subsystem/3(Isq)
  Merge1/1 -> iqmax/1
  Imaxsat/1 -> [Imax], Subtract/1
  [Imax] -> If Action Subsystem/4(maxI)

== system GridFormingConverter/Grid-Forming Converter/Grid-Forming Converter Control/Current Limiting/CurrentLimitingMethod/currentLimitAndVirtual/No Fault Ride Through ==
  Id : Inport
  Iq : Inport  Port=2
  Enable : EnablePort
  Constant{1..4} (4 alike) : Constant  Value=0
  Terminator : Terminator
  Terminator1 : Terminator
  delVd : Outport
  delVq : Outport  Port=2
  idmax : Outport  Port=3
  iqmax : Outport  Port=4
  wires:
  Constant3/1 -> iqmax/1
  Constant2/1 -> idmax/1
  Constant1/1 -> delVd/1
  Constant4/1 -> delVq/1
  Id/1 -> Terminator/1
  Iq/1 -> Terminator1/1

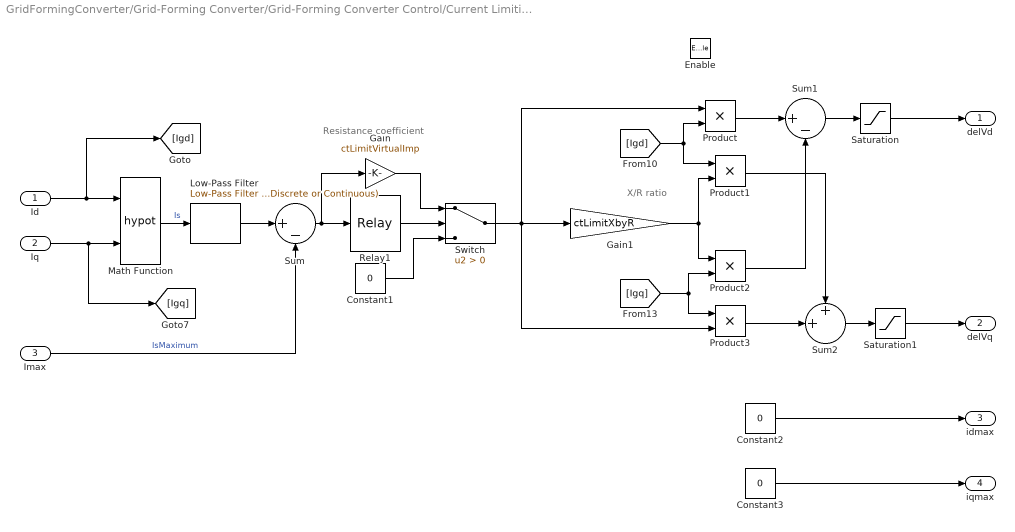
== system GridFormingConverter/Grid-Forming Converter/Grid-Forming Converter Control/Current Limiting/CurrentLimitingMethod/currentLimitAndVirtual/VI ==
  note: Resistance coefficient
  note: X/R ratio
  Id : Inport
  Iq : Inport  Port=2
  Imax : Inport  Port=3
  Enable : EnablePort
  Constant1 : Constant  Value=0
  Constant2 : Constant  Value=0
  Constant3 : Constant  Value=0
  Gain : Gain  Gain=ctLimitVirtualImp
  Gain1 : Gain  Gain=ctLimitXbyR
  Low-Pass Filter : eeGeneralControl/Low-Pass Filter (Discrete or Continuous)  K=1  T=currentVITimeConst  B=inf  A=-inf  init_option=Inherited from block input  x0=0  Ts=-1
  Math Function : Math  Operator=hypot
  Product{,1..3} (4 alike) : Product
  Relay1 : Relay  OnSwitchValue=0.01  OffSwitchValue=-0.1
  Saturation : Saturate  UpperLimit=1  LowerLimit=-1
  Saturation1 : Saturate  UpperLimit=1  LowerLimit=-1
  Sum : Sum  Inputs=|+-
  Sum1 : Sum  Inputs=|+-
  Sum2 : Sum  Inputs=++|
  Switch : Switch  Criteria=u2 > Threshold  SaturateOnIntegerOverflow=off  InputSameDT=off
  delVd : Outport
  delVq : Outport  Port=2
  idmax : Outport  Port=3
  iqmax : Outport  Port=4
  wires:
  Gain1/1 -> Product1/2, Product2/1
  Product3/1 -> Sum2/2
  Id/1 -> Math Function/1, [Igd]
  Sum2/1 -> Saturation1/1
  Sum/1 -> Gain/1, Relay1/1
  Sum1/1 -> Saturation/1
  Product/1 -> Sum1/1
  [Igq] -> Product3/1, Product2/2
  Iq/1 -> [Igq], Math Function/2
  Math Function/1 -> Low-Pass Filter/1  "Is"
  Switch/1 -> Product3/2, Product/1, Gain1/1
  [Igd] -> Product1/1, Product/2
  Saturation1/1 -> delVq/1
  Product1/1 -> Sum2/1
  Product2/1 -> Sum1/2
  Gain/1 -> Switch/1
  Constant1/1 -> Switch/3
  Saturation/1 -> delVd/1
  Constant3/1 -> iqmax/1
  Constant2/1 -> idmax/1
  Relay1/1 -> Switch/2
  Low-Pass Filter/1 -> Sum/1
  Imax/1 -> Sum/2  "IsMaximum"

== system GridFormingConverter/Grid-Forming Converter/Grid-Forming Converter Control/Current Limiting/CurrentLimitingMethod/currentSaturation/Compare ==
  u : Inport
  AND : Logic  IconShape=distinctive  AllPortsSameDT=off  OutDataTypeStr=boolean
  Compare To Constant : simulink/Logic and Bit Operations/Compare To Constant  relop=>  const=ctLimitDelayTime  OutDataTypeStr=boolean
  Data Type Conversion : DataTypeConversion  SaturateOnIntegerOverflow=off  RndMeth=Floor
  Data Type Conversion1 : DataTypeConversion  SaturateOnIntegerOverflow=off  RndMeth=Floor
  Discrete-Time Integrator : DiscreteIntegrator  IntegratorMethod=Integration: Backward Euler  ExternalReset=falling  SampleTime=currentControlTs  LimitOutput=on  UpperSaturationLimit=ctLimitDelayTime*2  LowerSaturationLimit=0  ICPrevOutput=DiscIntNeverNeededParam  ICPrevScaledInput=DiscIntNeverNeededParam
  Relay : Relay  OnSwitchValue=0.005*maxSatCurrentLimit  OffSwitchValue=-1*0.02*maxSatCurrentLimit
  Out1 : Outport
  wires:
  AND/1 -> Data Type Conversion/1
  Relay/1 -> Data Type Conversion1/1
  u/1 -> Relay/1
  Discrete-Time Integrator/1 -> Compare To Constant/1
  Data Type Conversion/1 -> Out1/1
  Data Type Conversion1/1 -> Discrete-Time Integrator/1, AND/1, Discrete-Time Integrator/2
  Compare To Constant/1 -> AND/2

== system GridFormingConverter/Grid-Forming Converter/Grid-Forming Converter Control/Current Limiting/CurrentLimitingMethod/currentSaturation/If Action Subsystem ==
  Is : Inport
  Isd : Inport  Port=2
  Isq : Inport  Port=3
  Action Port : ActionPort  ActionPortLabel=if(u1 > 0)
  Constant : Constant  Value=maxSatCurrentLimit
  Divide : Product  Inputs=*/
  Product : Product
  Product1 : Product
  Idmax : Outport
  Iqmax : Outport  Port=2
  wires:
  Constant/1 -> Divide/1
  Is/1 -> Divide/2
  Divide/1 -> Product1/2, Product/1
  Isd/1 -> Product1/1
  Isq/1 -> Product/2
  Product1/1 -> Idmax/1
  Product/1 -> Iqmax/1

== system GridFormingConverter/Grid-Forming Converter/Grid-Forming Converter Control/Current Limiting/CurrentLimitingMethod/currentSaturation/If Action Subsystem1 ==
  Action Port : ActionPort  ActionPortLabel=else
  Constant3 : Constant  Value=0
  Constant4 : Constant  Value=0
  Idmax : Outport
  Iqmax : Outport  Port=2
  wires:
  Constant4/1 -> Iqmax/1
  Constant3/1 -> Idmax/1

== system GridFormingConverter/Grid-Forming Converter/Grid-Forming Converter Control/Grid Voltage Reactive Power Support/Modifying Reactive Power Reference/Changing the Power Reference/ActivePowerReference ==
  note: Ensure Pref sign is maintained
  Id : Inport
  Vd : Inport  Port=2
  Pref : Inport  Port=3
  Abs1 : Abs  SaturateOnIntegerOverflow=off
  Abs2 : Abs  SaturateOnIntegerOverflow=off
  Min : MinMax  Inputs=2
  Product : Product
  Product2 : Product
  Saturation : Saturate  UpperLimit=1  LowerLimit=-1
  Sign : Signum
  PrefNew : Outport
  wires:
  Pref/1 -> Abs1/1, Sign/1
  Id/1 -> Product/1
  Sign/1 -> Product2/2
  Abs1/1 -> Min/2
  Product/1 -> Abs2/1
  Min/1 -> Product2/1
  Product2/1 -> Saturation/1
  Abs2/1 -> Min/1
  Vd/1 -> Product/2
  Saturation/1 -> PrefNew/1

== system GridFormingConverter/Grid-Forming Converter/Grid-Forming Converter Control/Grid Voltage Reactive Power Support/Modifying Reactive Power Reference/Changing the Power Reference/Estimate Id for Given Iq ==
  Iq : Inport
  Add Constant1 : Bias  Bias=1  SaturateOnIntegerOverflow=off
  Gain : Gain  Gain=-1
  Gain3 : Gain  Gain=0.9
  Sqrt : Sqrt
  Square : Math  Operator=square
  Id : Outport
  wires:
  Square/1 -> Gain/1
  Gain3/1 -> Id/1
  Gain/1 -> Add Constant1/1
  Sqrt/1 -> Gain3/1
  Add Constant1/1 -> Sqrt/1
  Iq/1 -> Square/1

== system GridFormingConverter/Grid-Forming Converter/Grid-Forming Converter Control/Grid Voltage Reactive Power Support/Modifying Reactive Power Reference/Changing the Power Reference/EstimateIqForReactivePower ==
  note: Computing minimum reactive current as per GC0137
  Vmin : Inport
  Vd : Inport  Port=2
  Vs : Inport  Port=3
  Abs : Abs  SaturateOnIntegerOverflow=off
  Add : Sum
  Add Constant : Bias  Bias=1  SaturateOnIntegerOverflow=off
  GC0137 line slope : Gain  Gain=-1.4578
  Low Voltage Support : Subsystem
  Saturation : Saturate  UpperLimit=1  LowerLimit=0
  Iq : Outport
  wires:
  Abs/1 -> GC0137 line slope/1
  GC0137 line slope/1 -> Add Constant/1
  Vs/1 -> Abs/1
  Add/1 -> Saturation/1
  Saturation/1 -> Iq/1
  Add Constant/1 -> Add/2
  Vmin/1 -> Low Voltage Support/1(Vin)
  Vd/1 -> Low Voltage Support/2(Vd)
  Low Voltage Support/1(Iqsupport) -> Add/1

== system GridFormingConverter/Grid-Forming Converter/Grid-Forming Converter Control/Grid Voltage Reactive Power Support/Modifying Reactive Power Reference/Changing the Power Reference/ReactivePowerReference ==
  Vd : Inport
  Iq : Inport  Port=2
  Compute Power : Product
  Constant : Constant  Value=0.3
  Gain2 : Gain  Gain=1.05
  Switch : Switch  Criteria=u2 > Threshold  Threshold=0.3  SaturateOnIntegerOverflow=off  InputSameDT=off
  QrefNew : Outport
  wires:
  Compute Power/1 -> QrefNew/1
  Gain2/1 -> Compute Power/2
  Constant/1 -> Switch/3
  Iq/1 -> Gain2/1
  Vd/1 -> Switch/2, Switch/1
  Switch/1 -> Compute Power/1
